simulink model "DuongDucQuan_20001967"  (R2016a)
settings: Solver=ode45  StartTime=0.0  StopTime=10.0  RelTol=1e-3
settings Model: Creator=Quandeptrai  LastModifiedBy=Quandeptrai

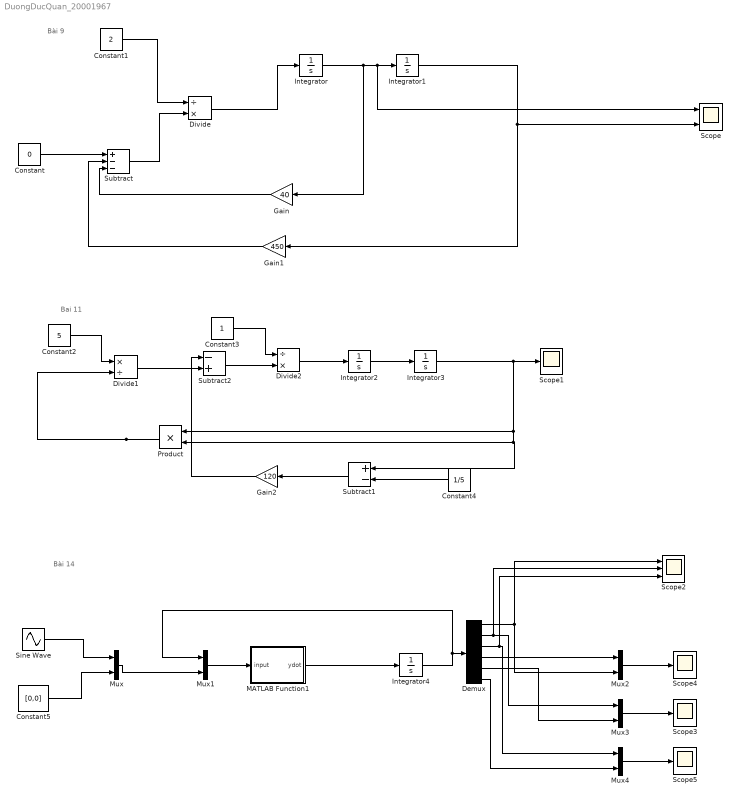
== system DuongDucQuan_20001967 ==
  note: Bài 14
  note: Bai 11
  note: Bài 9
  Constant : Constant  Value=0
  Constant1 : Constant  Value=2
  Constant2 : Constant  Value=5
  Constant3 : Constant
  Constant4 : Constant  Value=1/5
  Constant5 : Constant  Value=[0,0]
  Demux : Demux  Outputs=6
  Divide : Product  Inputs=/*
  Divide1 : Product  Inputs=*/
  Divide2 : Product  Inputs=/*
  Gain : Gain  Gain=40
  Gain1 : Gain  Gain=450
  Gain2 : Gain  Gain=120
  Integrator : Integrator
  Integrator1 : Integrator  InitialCondition=0.01
  Integrator2 : Integrator
  Integrator3 : Integrator  InitialCondition=0.2
  Integrator4 : Integrator  InitialCondition=[0;0;0;0;0;0]
  MATLAB Function1 : MATLAB Function  TreatAsAtomicUnit=on
  Mux{,1..4} (5 alike) : Mux  Inputs=2
  Product : Product
  Scope : Scope  NumInputPorts=2
  Scope{1,3..5} (4 alike) : Scope
  Scope2 : Scope  NumInputPorts=3
  Sine Wave : Sin  Amplitude=5  Frequency=10  SampleTime=0
  Subtract : Sum  Inputs=+--
  Subtract1 : Sum  Inputs=+-
  Subtract2 : Sum  Inputs=-+
  wires:
  Constant1/1 -> Divide/1
  Constant/1 -> Subtract/1
  Subtract/1 -> Divide/2
  Divide/1 -> Integrator/1
  Integrator/1 -> Scope/1, Integrator1/1, Gain/1
  Gain/1 -> Subtract/3
  Gain1/1 -> Subtract/2
  Integrator1/1 -> Gain1/1, Scope/2
  Constant3/1 -> Divide2/1
  Divide1/1 -> Subtract2/2
  Subtract2/1 -> Divide2/2
  Divide2/1 -> Integrator2/1
  Integrator2/1 -> Integrator3/1
  Integrator3/1 -> Scope1/1, Subtract1/1, Product/2, Product/1
  Constant4/1 -> Subtract1/2
  Product/1 -> Divide1/2
  Constant2/1 -> Divide1/1
  Subtract1/1 -> Gain2/1
  Gain2/1 -> Subtract2/1
  Mux/1 -> Mux1/2
  Mux1/1 -> MATLAB Function1/1(input)
  MATLAB Function1/1(ydot) -> Integrator4/1
  Integrator4/1 -> Mux1/1, Demux/1
  Demux/1 -> Mux2/2, Scope2/1
  Demux/2 -> Scope2/2, Mux3/1
  Demux/3 -> Scope2/3, Mux4/1
  Demux/6 -> Mux4/2
  Demux/5 -> Mux3/2
  Demux/4 -> Mux2/1
  Mux4/1 -> Scope5/1
  Mux2/1 -> Scope4/1
  Mux3/1 -> Scope3/1
  Sine Wave/1 -> Mux/1
  Constant5/1 -> Mux/2

== matlab function DuongDucQuan_20001967/MATLAB Function1 ==
  data: input input; ydot output
function ydot = fcn(input)
q1=input(1); q2=input(2);q3=input(3); q1_dot=input(4); q2_dot=input(5); q3_dot=input(6);
q = [q1;q2;q3];

u1=input(7); u2=input(8); u3=input(9); u=[u1; u2; u3];
M = [12, 0, 0; 0, 15, 0; 0, 0, 20];

B = [1000, -1000, 0;-1000, 2000, -1000;0, -1000, 1000];
C = [10 -10 0;-10 20 -10;0 -10 10];
gq= C*q;

q_dot=[q1_dot; q2_dot; q3_dot];
q_2dot= M\(u - B*q_dot - gq);
ydot=[q_dot; q_2dot];
